simulink model "pneumaticClutchSoln"  (R2017b)
settings: Solver=ode23t  StartTime=0.0  StopTime=10.0  RelTol=1e-3  AbsTol=1e-3  EnableMultiTasking=on
libraries: fl_lib x8, Pneumatic_lib x6, nesl_utility x5, sdl_lib x1
settings Model: Creator=scastro  LastModifiedBy=chahn
settings DataIOCC: LimitDataPoints=on  SaveFormat=Array
settings OptimizationCC: LifeSpan=inf
settings DebuggingCC: SFUnexpectedBacktrackingDiag=warning  SFNoUnconditionalDefaultTransitionDiag=warning  SFExecutionAtInitializationDiag=none
settings HardwareCC: ProdBitPerPointer=32  ProdBitPerSizeT=32  ProdBitPerPtrDiffT=32  ProdLargestAtomicFloat=None  ProdIntDivRoundTo=Undefined  ProdEndianess=Unspecified  ProdWordSize=32  ProdHWDeviceType=32-bit Generic
settings ModelReferenceCC: PropagateSignalLabelsOutOfModel=off
settings CodeAppCC: StateflowObjectComments=on
settings GRTTargetCC: TargetLangStandard=C89/C90 (ANSI)  GeneratePreprocessorConditionals=Disable all
settings ConfigComp: CovMetricSettings=dw  CovHtmlReporting=on  CovSaveCumulativeToWorkspaceVar=on  CovSaveSingleToWorkspaceVar=on  CovExternalEMLEnable=off
settings SimscapeCC: SimscapeNormalizeSystem=off  SimscapeLogType=all  SimscapeLogDataHistory=10000

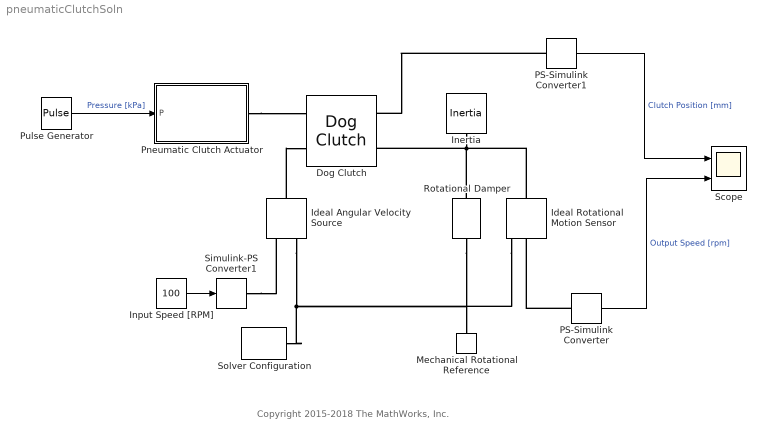
== system pneumaticClutchSoln ==
  note: Copyright 2015-2018 The MathWorks, Inc.
  Dog Clutch : sdl_lib/Clutches/Dog Clutch  model=1  max_torque=1000 N*m  n_teeth=6  clutch_backlash=10 deg  tooth_height=10 mm  radius=50 mm  back_stop=1  ring_hub_gap=3 mm  clutch_stiffness=1e+7 N*m/rad  clutch_damping=100 N*m/(rad/s)  transl_stiffness=1e+6 N/m  transl_damping=1000 N/(m/s)  visc_fric_transl=100 N/(m/s)  fric_coeff=0.05  direction=1  engagement_velocity=Inf rad/s  engagement_overlap=5 mm  initial_state_engaged=0  init_pos=0 mm  init_rel_angle=0 deg  temperature_TLU=[280, 300, 320] K  max_torque_vector=[1000, 1050, 1000] N*m  interp_method=1  extrap_method=1  thermal_mass=25 kJ/K  T_init=300 K
      settings: SourceProductName=Simscape Driveline  SourceProductBaseCode=LD
  Ideal Angular Velocity Source : fl_lib/Mechanical/Mechanical Sources/Ideal Angular Velocity Source
  Ideal Rotational Motion Sensor : fl_lib/Mechanical/Mechanical Sensors/Ideal Rotational Motion Sensor  offset=0 rad
  Inertia : fl_lib/Mechanical/Rotational Elements/Inertia  inertia=0.1 kg*m^2  w_specify=off  w_priority=High  w=0 rad/s  w_nominal_specify=off  w_nominal_unit=rad/s  w_nominal_value=1  t_specify=off  t_priority=High  t=0 N*m  t_nominal_specify=off  t_nominal_unit=N*m  t_nominal_value=1
  Input Speed [RPM] : Constant  Value=100
  Mechanical Rotational Reference : fl_lib/Mechanical/Rotational Elements/Mechanical Rotational Reference
  PS-Simulink Converter : nesl_utility/PS-Simulink Converter  PhysicalDomain=network_engine_domain  SubClassName=ps_output  LeftPortType=input  RightPortType=output  PseudoPeriodic=off  Frequencies=[]  Unit=rpm  AffineConversion=off
  PS-Simulink Converter1 : nesl_utility/PS-Simulink Converter  PhysicalDomain=network_engine_domain  SubClassName=ps_output  LeftPortType=input  RightPortType=output  PseudoPeriodic=off  Frequencies=[]  Unit=mm  AffineConversion=off
  Pneumatic Clutch Actuator : Subsystem
  Pulse Generator : DiscretePulseGenerator  PulseType=Time based  Period=3  PulseWidth=50
  Rotational Damper : fl_lib/Mechanical/Rotational Elements/Rotational Damper  D=0.5 N*m/(rad/s)  w_specify=off  w_priority=High  w=0 rad/s  w_nominal_specify=off  w_nominal_unit=rad/s  w_nominal_value=1  t_specify=off  t_priority=High  t=0 N*m  t_nominal_specify=off  t_nominal_unit=N*m  t_nominal_value=1
  Scope : Scope  NumInputPorts=2
  Simulink-PS Converter1 : nesl_utility/Simulink-PS Converter  PhysicalDomain=network_engine_domain  SubClassName=ps_input  LeftPortType=input  RightPortType=output  PseudoPeriodic=off  Frequencies=[]  NoiseDistribution=none  NoiseParameters=[]  Unit=rpm  AffineConversion=off  FilteringAndDerivatives=zero  SimscapeFilterOrder=1  InputFilterTimeConstant=0.001  UdotUserProvided=1
  Solver Configuration : nesl_utility/Solver Configuration  PhysicalDomain=network_engine_domain  SubClassName=solver  LeftPortType=input  RightPortType=generic  Accelerate=off  Tones=[]  Harmonics=[]  SimulateNoise=off  Profile=off  UseLocalSampling=off  EnableSwitchedLinearOptims=on  FrequencyDomain=off  UseCCode=off  RelTol=0.001  AbsTol=1e-06  MinStep=1e-09  ToWorkspace=off  RevertToSquareIcSolve=off  NumHomotopyIterations=100  PhasorMode=off  PhasorModeNumHarmonics=1  DoDC=off  ResidualTolerance=1e-09  UseLocalSolver=off  LocalSolverChoice=NE_BACKWARD_EULER_ADVANCER  LocalSolverSampleTime=0.001  DoFixedCost=off  MaxNonlinIter=3  MaxModeIter=2  LinearAlgebra=Sparse  DelaysMemoryBudget=1024  AutomaticFiltering=on  FilteringTimeConstant=0.001
  wires:
  PS-Simulink Converter/1 -> Scope/2  "Output Speed [rpm]"
  Input Speed [RPM]/1 -> Simulink-PS Converter1/1
  PS-Simulink Converter1/1 -> Scope/1  "Clutch Position [mm]"
  Pulse Generator/1 -> Pneumatic Clutch Actuator/1(P)  "Pressure [kPa]"
  connections:
  Ideal Angular Velocity Source/LConn1 -- Dog Clutch/LConn2
  Ideal Angular Velocity Source/RConn2 -- Ideal Rotational Motion Sensor/RConn1 -- Mechanical Rotational Reference/LConn1 -- Rotational Damper/RConn1 -- Solver Configuration/RConn1
  Simulink-PS Converter1/RConn1 -- Ideal Angular Velocity Source/RConn1
  Inertia/LConn1 -- Ideal Rotational Motion Sensor/LConn1 -- Rotational Damper/LConn1 -- Dog Clutch/RConn2
  PS-Simulink Converter/LConn1 -- Ideal Rotational Motion Sensor/RConn2
  PS-Simulink Converter1/LConn1 -- Dog Clutch/RConn1
  Pneumatic Clutch Actuator/RConn1 -- Dog Clutch/LConn1

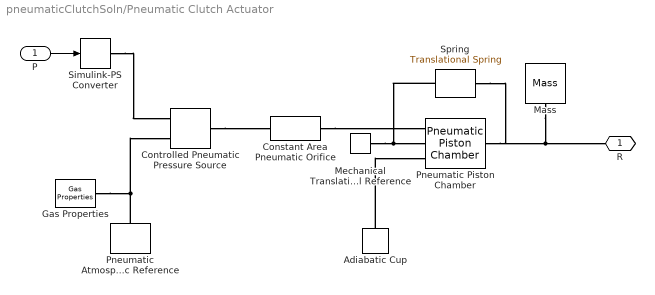
== system pneumaticClutchSoln/Pneumatic Clutch Actuator ==
  P : Inport
  Adiabatic Cup : Pneumatic_lib/Pneumatic Elements/Adiabatic Cup
  Constant Area Pneumatic Orifice : Pneumatic_lib/Pneumatic Elements/Constant Area Pneumatic Orifice  Cd=0.82  Area=5e-5 m^2  G_specify=off  G_priority=High  G=0 kg/s  G_nominal_specify=off  G_nominal_unit=kg/s  G_nominal_value=1  Q1_specify=off  Q1_priority=High  Q1=0 J/s  Q1_nominal_specify=off  Q1_nominal_unit=J/s  Q1_nominal_value=1  Q2_specify=off  Q2_priority=High  Q2=0 J/s  Q2_nominal_specify=off  Q2_nominal_unit=J/s  Q2_nominal_value=1  p1_specify=off  p1_priority=High  p1=1e+5 Pa  p1_nominal_specify=off  p1_nominal_unit=Pa  p1_nominal_value=1  p2_specify=off  p2_priority=High  p2=1e+5 Pa  p2_nominal_specify=off  p2_nominal_unit=Pa  p2_nominal_value=1  T1_specify=off  T1_priority=High  T1=300 K  T1_nominal_specify=off  T1_nominal_unit=K  T1_nominal_value=1  T2_specify=off  T2_priority=High  T2=300 K  T2_nominal_specify=off  T2_nominal_unit=K  T2_nominal_value=1
  Controlled Pneumatic Pressure Source : Pneumatic_lib/Pneumatic Sources/Controlled Pneumatic Pressure Source
  Gas Properties : Pneumatic_lib/Pneumatic Utilities/Gas Properties  c_p=1005 J/kg/K  c_v=717.95 J/kg/K  viscosity=18.21e-6 s*Pa  Pa=101325 Pa  Ta=293.15 K  range_error=2
  Mass : fl_lib/Mechanical/Translational Elements/Mass  mass=0.1 kg  v_specify=off  v_priority=High  v=0 m/s  v_nominal_specify=off  v_nominal_unit=m/s  v_nominal_value=1  f_specify=off  f_priority=High  f=0 N  f_nominal_specify=off  f_nominal_unit=N  f_nominal_value=1
  Mechanical Translational Reference : fl_lib/Mechanical/Translational Elements/Mechanical Translational Reference
  Pneumatic Atmospheric Reference : Pneumatic_lib/Pneumatic Elements/Pneumatic Atmospheric Reference
  Pneumatic Piston Chamber : Pneumatic_lib/Pneumatic Elements/Pneumatic Piston Chamber  Area=2.5e-3 m^2  x0=0 m  V0=1e-5 m^3  or=1  pressure_specify=off  pressure_priority=High  pressure=1e+5 Pa  pressure_nominal_specify=off  pressure_nominal_unit=Pa  pressure_nominal_value=1  temperature_specify=off  temperature_priority=High  temperature=300 K  temperature_nominal_specify=off  temperature_nominal_unit=K  temperature_nominal_value=1  gas_flow_specify=off  gas_flow_priority=High  gas_flow=0 kg/s  gas_flow_nominal_specify=off  gas_flow_nominal_unit=kg/s  gas_flow_nominal_value=1  heat_flow_specify=off  heat_flow_priority=High  heat_flow=0 J/s  heat_flow_nominal_specify=off  heat_flow_nominal_unit=J/s  heat_flow_nominal_value=1  heat_exch_flow_specify=off  heat_exch_flow_priority=High  heat_exch_flow=0 J/s  heat_exch_flow_nominal_specify=off  heat_exch_flow_nominal_unit=J/s  heat_exch_flow_nominal_value=1  velocity_specify=off  velocity_priority=High  velocity=0 m/s  velocity_nominal_specify=off  velocity_nominal_unit=m/s  velocity_nominal_value=1  force_specify=off  force_priority=High  force=0 N  force_nominal_specify=off  force_nominal_unit=N  force_nominal_value=1
  Simulink-PS Converter : nesl_utility/Simulink-PS Converter  PhysicalDomain=network_engine_domain  SubClassName=ps_input  LeftPortType=input  RightPortType=output  PseudoPeriodic=off  Frequencies=[]  NoiseDistribution=none  NoiseParameters=[]  Unit=kPa  AffineConversion=off  FilteringAndDerivatives=zero  SimscapeFilterOrder=1  InputFilterTimeConstant=0.001  UdotUserProvided=1
  Spring : fl_lib/Mechanical/Translational Elements/Translational Spring  spr_rate=250 N/m  v_specify=off  v_priority=High  v=0 m/s  v_nominal_specify=off  v_nominal_unit=m/s  v_nominal_value=1  f_specify=off  f_priority=High  f=0 N  f_nominal_specify=off  f_nominal_unit=N  f_nominal_value=1  x_specify=off  x_priority=High  x=0 m  x_nominal_specify=off  x_nominal_unit=m  x_nominal_value=1
  R : PMIOPort  Port=1  Side=Right
  wires:
  P/1 -> Simulink-PS Converter/1
  connections:
  Mechanical Translational Reference/LConn1 -- Spring/RConn1 -- Pneumatic Piston Chamber/LConn2
  Constant Area Pneumatic Orifice/RConn1 -- Pneumatic Piston Chamber/LConn1
  Simulink-PS Converter/RConn1 -- Controlled Pneumatic Pressure Source/RConn2
  Controlled Pneumatic Pressure Source/LConn1 -- Constant Area Pneumatic Orifice/LConn1
  Pneumatic Atmospheric Reference/LConn1 -- Gas Properties/RConn1 -- Controlled Pneumatic Pressure Source/RConn1
  Mass/LConn1 -- R/RConn1 -- Spring/LConn1 -- Pneumatic Piston Chamber/RConn1
  Adiabatic Cup/LConn1 -- Pneumatic Piston Chamber/LConn3
